simulink model "zadatak2"  (R2016b)
settings: Solver=VariableStepAuto  StartTime=0.0  StopTime=30  FixedStep=0.0001  RelTol=1e-3
settings Model: Creator=Luka  LastModifiedBy=Luka

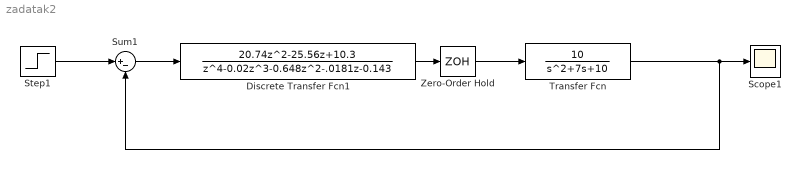
== system zadatak2 ==
  Discrete Transfer Fcn1 : DiscreteTransferFcn  Numerator=[20.74 -25.56 10.3]  Denominator=[1 -0.02 -0.648 -.0181 -0.143]
  Scope1 : Scope
  Step1 : Step  Time=0  SampleTime=0
  Sum1 : Sum  Inputs=|+-
  Transfer Fcn : TransferFcn  Numerator=[10]  Denominator=[1 7 10]
  Zero-Order Hold : ZeroOrderHold  SampleTime=0.1
  wires:
  Step1/1 -> Sum1/1
  Sum1/1 -> Discrete Transfer Fcn1/1
  Discrete Transfer Fcn1/1 -> Zero-Order Hold/1
  Transfer Fcn/1 -> Sum1/2, Scope1/1
  Zero-Order Hold/1 -> Transfer Fcn/1
